simulink model "robot_4DOF_jointspace"  (Simulink 7.3)
settings: Solver=ode4  StartTime=0.0  StopTime=5  FixedStep=.002  MinStep=.002  RelTol=1e-3
libraries: simulink_extras x1, dspinverses x1
(part 1 of 2)
settings Model: Creator=arash  LastModifiedBy=arash
settings SolverCC: ExtrapolationOrder=1

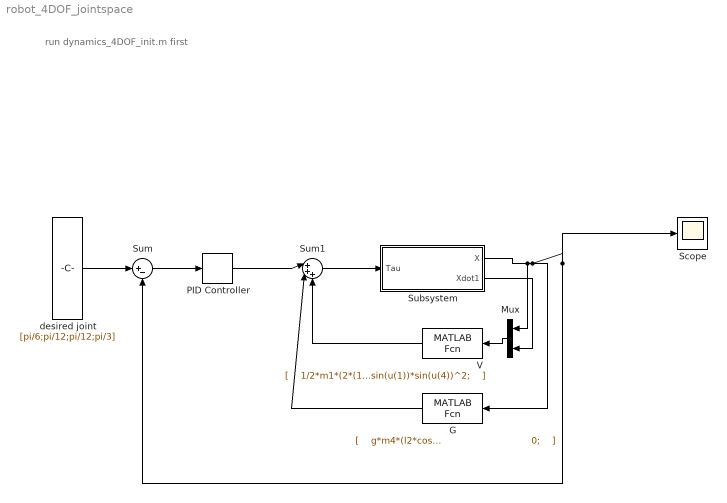
== system robot_4DOF_jointspace ==
  note: run dynamics_4DOF_init.m first
  G : MATLABFcn  MATLABFcn=|  OutputDimensions=4  OutputSignalType=real  Output1D=off
      | [
      |  
      |  g*m4*(l2*cos(u(1) + u(2)) + l1*cos(u(1)) + 1/2*l3*cos(u(1) + u(2) + u(3))) + g*m3*(1/2*l2*cos(u(1) + u(2)) + l1*cos(u(1))) + 1/2*g*l1*m2*cos(u(1));
      |                                                          g*m4*(l2*cos(u(1) + u(2)) + 1/2*l3*cos(u(1) + u(2) + u(3))) + 1/2*g*l2*m3*cos(u(1) + u(2));
      |                                                                                                                 1/2*g*l3*m4*cos(u(1) + u(2) + u(3));
      |                                                                                                                                                   0;
      |  
      |  ]
  Mux : Mux  Inputs=2
  PID Controller : simulink_extras/Additional Linear/PID Controller  SystemSampleTime=-1  P=[60;50;40;40]*10  I=[0;0;0;0]  D=[10;7;7;6]*5
  Scope : Scope
      settings: YMin=-0.05  YMax=1.1
  Subsystem : Subsystem
  Sum : Sum  Inputs=|+-  OutDataType=fixdt(1, 16)  OutScaling=2^0
  Sum1 : Sum  Inputs=|+++  OutDataType=fixdt(1, 16)  OutScaling=2^0
  V : MATLABFcn  MATLABFcn=|  OutputDimensions=4  OutputSignalType=real  Output1D=off
      | [
      |  
      |  1/2*m1*(2*(1/2*l1*u(8)*sin(u(1))*sin(u(4)) - 1/2*l1*u(5)*cos(u(1))*cos(u(4)))*(1/2*l1*u(5)*cos(u(4))*sin(u(1)) + 1/2*l1*u(8)*cos(u(1))*sin(u(4))) - 2*(1/2*l1*u(5)*sin(u(1))*sin(u(4)) - 1/2*l1*u(8)*cos(u(1))*cos(u(4)))*(1/2*l1*u(5)*cos(u(1))*sin(u(4)) + 1/2*l1*u(8)*cos(u(4))*sin(u(1))) + 1/2*l1^2*u(5)^2*cos(u(1))*sin(u(1))) + 1/2*m2*(2*sin(u(4))*(1/2*l2*sin(u(1) + u(2)) + l1*sin(u(1)))*(sin(u(4))*(1/2*l2*cos(u(1) + u(2)) + l1*cos(u(1)))*u(8)^2 + 2*cos(u(4))*(l1*u(5)*sin(u(1)) + 1/2*l2*sin(u(1) + u(2))*(u(5) + u(6)))*u(8) + sin(u(4))*(1/2*l2*cos(u(1) + u(2))*(u(5) + u(6))^2 + l1*u(5)^2*cos(u(1)))) - 2*(1/2*l2*sin(u(1) + u(2))*(u(5) + u(6))^2 + l1*u(5)^2*sin(u(1)))*(1/2*l2*cos(u(1) + u(2)) + l1*cos(u(1))) - 2*(l1*u(5)*cos(u(1)) + 1/2*l2*cos(u(1) + u(2))*(u(5) + u(6)))*(l1*u(5)*sin(u(1)) + 1/2*l2*sin(u(1) + u(2))*(u(5) + u(6))) + 2*cos(u(4))*(cos(u(4))*(l1*u(5)*sin(u(1)) + 1/2*l2*sin(u(1) + u(2))*(u(5) + u(6))) + u(8)*sin(u(4))*(1/2*l2*cos(u(1) + u(2)) + l1*cos(u(1))))*(l1*u(5)*cos(u(1)) + 1/2*l2*cos(u(1) + u(2))*(u(5) + u(6))) + 2*sin(u(4))*(sin(u(4))*(l1*u(5)*sin(u(1)) + 1/2*l2*sin(u(1) + u(2))*(u(5) + u(6))) - u(8)*cos(u(4))*(1/2*l2*cos(u(1) + u(2)) + l1*cos(u(1))))*(l1*u(5)*cos(u(1)) + 1/2*l2*cos(u(1) + u(2))*(u(5) + u(6))) + 2*cos(u(4))*(1/2*l2*sin(u(1) + u(2)) + l1*sin(u(1)))*(cos(u(4))*(1/2*l2*cos(u(1) + u(2)) + l1*cos(u(1)))*u(8)^2 - 2*sin(u(4))*(l1*u(5)*sin(u(1)) + 1/2*l2*sin(u(1) + u(2))*(u(5) + u(6)))*u(8) + cos(u(4))*(1/2*l2*cos(u(1) + u(2))*(u(5) + u(6))^2 + l1*u(5)^2*cos(u(1)))) + 2*u(8)*cos(u(4))*(sin(u(4))*(l1*u(5)*sin(u(1)) + 1/2*l2*sin(u(1) + u(2))*(u(5) + u(6))) - u(8)*cos(u(4))*(1/2*l2*cos(u(1) + u(2)) + l1*cos(u(1))))*(1/2*l2*sin(u(1) + u(2)) + l1*sin(u(1))) - 2*u(8)*sin(u(4))*(cos(u(4))*(l1*u(5)*sin(u(1)) + 1/2*l2*sin(u(1) + u(2))*(u(5) + u(6))) + u(8)*sin(u(4))*(1/2*l2*cos(u(1) + u(2)) + l1*cos(u(1))))*(1/2*l2*sin(u(1) + u(2)) + l1*sin(u(1)))) + c1*u(5) - 1/2*m3*(2*(sin(u(4))*(l1*u(5)*cos(u(1)) + 1/2*l3*cos(u(1) + u(2) + u(3))*(u(5) + u(6) + u(7)) + l2*cos(u(1) + u(2))*(u(5) + u(6))) + u(8)*cos(u(4))*(l2*sin(u(1) + u(2)) + l1*sin(u(1)) + 1/2*l3*sin(u(1) + u(2) + u(3))))*(sin(u(4))*(l1*u(5)*sin(u(1)) + 1/2*l3*sin(u(1) + u(2) + u(3))*(u(5) + u(6) + u(7)) + l2*sin(u(1) + u(2))*(u(5) + u(6))) - u(8)*cos(u(4))*(l2*cos(u(1) + u(2)) + l1*cos(u(1)) + 1/2*l3*cos(u(1) + u(2) + u(3)))) - 2*(l1*u(5)*sin(u(1)) + 1/2*l3*sin(u(1) + u(2) + u(3))*(u(5) + u(6) + u(7)) + l2*sin(u(1) + u(2))*(u(5) + u(6)))*(l1*u(5)*cos(u(1)) + 1/2*l3*cos(u(1) + u(2) + u(3))*(u(5) + u(6) + u(7)) + l2*cos(u(1) + u(2))*(u(5) + u(6))) + 2*(cos(u(4))*(l1*u(5)*sin(u(1)) + 1/2*l3*sin(u(1) + u(2) + u(3))*(u(5) + u(6) + u(7)) + l2*sin(u(1) + u(2))*(u(5) + u(6))) + u(8)*sin(u(4))*(l2*cos(u(1) + u(2)) + l1*cos(u(1)) + 1/2*l3*cos(u(1) + u(2) + u(3))))*(cos(u(4))*(l1*u(5)*cos(u(1)) + 1/2*l3*cos(u(1) + u(2) + u(3))*(u(5) + u(6) + u(7)) + l2*cos(u(1) + u(2))*(u(5) + u(6))) - u(8)*sin(u(4))*(l2*sin(u(1) + u(2)) + l1*sin(u(1)) + 1/2*l3*sin(u(1) + u(2) + u(3))))) - 1/2*m2*(2*(sin(u(4))*(l1*u(5)*cos(u(1)) + 1/2*l2*cos(u(1) + u(2))*(u(5) + u(6))) + u(8)*cos(u(4))*(1/2*l2*sin(u(1) + u(2)) + l1*sin(u(1))))*(sin(u(4))*(l1*u(5)*sin(u(1)) + 1/2*l2*sin(u(1) + u(2))*(u(5) + u(6))) - u(8)*cos(u(4))*(1/2*l2*cos(u(1) + u(2)) + l1*cos(u(1)))) + 2*(cos(u(4))*(l1*u(5)*sin(u(1)) + 1/2*l2*sin(u(1) + u(2))*(u(5) + u(6))) + u(8)*sin(u(4))*(1/2*l2*cos(u(1) + u(2)) + l1*cos(u(1))))*(cos(u(4))*(l1*u(5)*cos(u(1)) + 1/2*l2*cos(u(1) + u(2))*(u(5) + u(6))) - u(8)*sin(u(4))*(1/2*l2*sin(u(1) + u(2)) + l1*sin(u(1)))) - 2*(l1*u(5)*cos(u(1)) + 1/2*l2*cos(u(1) + u(2))*(u(5) + u(6)))*(l1*u(5)*sin(u(1)) + 1/2*l2*sin(u(1) + u(2))*(u(5) + u(6)))) + 1/2*m3*(2*cos(u(4))*(l2*sin(u(1) + u(2)) + l1*sin(u(1)) + 1/2*l3*sin(u(1) + u(2) + u(3)))*(cos(u(4))*(l2*cos(u(1) + u(2)) + l1*cos(u(1)) + 1/2*l3*cos(u(1) + u(2) + u(3)))*u(8)^2 - 2*sin(u(4))*(l1*u(5)*sin(u(1)) + 1/2*l3*sin(u(1) + u(2) + u(3))*(u(5) + u(6) + u(7)) + l2*sin(u(1) + u(2))*(u(5) + u(6)))*u(8) + cos(u(4))*(1/2*l3*cos(u(1) + u(2) + u(3))*(u(5) + u(6) + u(7))^2 + l2*cos(u(1) + u(2))*(u(5) + u(6))^2 + l1*u(5)^2*cos(u(1)))) - 2*(1/2*l3*sin(u(1) + u(2) + u(3))*(u(5) + u(6) + u(7))^2 + l2*sin(u(1) + u(2))*(u(5) + u(6))^2 + l1*u(5)^2*sin(u(1)))*(l2*cos(u(1) + u(2)) + l1*cos(u(1)) + 1/2*l3*cos(u(1) + u(2) + u(3))) - 2*(l1*u(5)*sin(u(1)) + 1/2*l3*sin(u(1) + u(2) + u(3))*(u(5) + u(6) + u(7)) + l2*sin(u(1) + u(2))*(u(5) + u(6)))*(l1*u(5)*cos(u(1)) + 1/2*l3*cos(u(1) + u(2) + u(3))*(u(5) + u(6) + u(7)) + l2*cos(u(1) + u(2))*(u(5) + u(6))) + 2*sin(u(4))*(l2*sin(u(1) + u(2)) + l1*sin(u(1)) + 1/2*l3*sin(u(1) + u(2) + u(3)))*(sin(u(4))*(l2*cos(u(1) + u(2)) + l1*cos(u(1)) + 1/2*l3*cos(u(1) + u(2) + u(3)))*u(8)^2 + 2*cos(u(4))*(l1*u(5)*sin(u(1)) + 1/2*l3*sin(u(1) + u(2) + u(3))*(u(5) + u(6) + u(7)) + l2*sin(u(1) + u(2))*(u(5) + u(6)))*u(8) + sin(u(4))*(1/2*l3*cos(u(1) + u(2) + u(3))*(u(5) + u(6) + u(7))^2 + l2*cos(u(1) + u(2))*(u(5) + u(6))^2 + l1*u(5)^2*cos(u(1)))) + 2*cos(u(4))*(cos(u(4))*(l1*u(5)*sin(u(1)) + 1/2*l3*sin(u(1) + u(2) + u(3))*(u(5) + u(6) + u(7)) + l2*sin(u(1) + u(2))*(u(5) + u(6))) + u(8)*sin(u(4))*(l2*cos(u(1) + u(2)) + l1*cos(u(1)) + 1/2*l3*cos(u(1) + u(2) + u(3))))*(l1*u(5)*cos(u(1)) + 1/2*l3*cos(u(1) + u(2) + u(3))*(u(5) + u(6) + u(7)) + l2*cos(u(1) + u(2))*(u(5) + u(6))) + 2*sin(u(4))*(sin(u(4))*(l1*u(5)*sin(u(1)) + 1/2*l3*sin(u(1) + u(2) + u(3))*(u(5) + u(6) + u(7)) + l2*sin(u(1) + u(2))*(u(5) + u(6))) - u(8)*cos(u(4))*(l2*cos(u(1) + u(2)) + l1*cos(u(1)) + 1/2*l3*cos(u(1) + u(2) + u(3))))*(l1*u(5)*cos(u(1)) + 1/2*l3*cos(u(1) + u(2) + u(3))*(u(5) + u(6) + u(7)) + l2*cos(u(1) + u(2))*(u(5) + u(6))) + 2*u(8)*cos(u(4))*(sin(u(4))*(l1*u(5)*sin(u(1)) + 1/2*l3*sin(u(1) + u(2) + u(3))*(u(5) + u(6) + u(7)) + l2*sin(u(1) + u(2))*(u(5) + u(6))) - u(8)*cos(u(4))*(l2*cos(u(1) + u(2)) + l1*cos(u(1)) + 1/2*l3*cos(u(1) + u(2) + u(3))))*(l2*sin(u(1) + u(2)) + l1*sin(u(1)) + 1/2*l3*sin(u(1) + u(2) + u(3))) - 2*u(8)*sin(u(4))*(cos(u(4))*(l1*u(5)*sin(u(1)) + 1/2*l3*sin(u(1) + u(2) + u(3))*(u(5) + u(6) + u(7)) + l2*sin(u(1) + u(2))*(u(5) + u(6))) + u(8)*sin(u(4))*(l2*cos(u(1) + u(2)) + l1*cos(u(1)) + 1/2*l3*cos(u(1) + u(2) + u(3))))*(l2*sin(u(1) + u(2)) + l1*sin(u(1)) + 1/2*l3*sin(u(1) + u(2) + u(3)))) + Ixx1*u(8)^2*cos(u(1))*sin(u(1)) - Izz1*u(8)^2*cos(u(1))*sin(u(1)) + Ixx3*u(8)^2*cos(u(1) + u(2) + u(3))*sin(u(1) + u(2) + u(3)) - Izz3*u(8)^2*cos(u(1) + u(2) + u(3))*sin(u(1) + u(2) + u(3)) + Ixx2*u(8)^2*cos(u(1) + u(2))*sin(u(1) + u(2)) - Izz2*u(8)^2*cos(u(1) + u(2))*sin(u(1) + u(2));
      |                                                                                                                                                                                                                                                                                                                                                                                                                                                                                                                                                                                                                                                                                                                                                                                                                                                                                                                                                                                                                                                                                                                                                                                                                                                                                                                                                                                                                                                                                                                                                                                                                                                                                                                                                                                                                                                                                                                                                                                                                                                                                                                                                                                                                                                                                                                                                                                                                                                                                                                                                                                                                                                                                                                                                                                                                                                                                                                                                                                                                                                                                                                                                                                                                                                                                                                                                                                                                                                                                                                                                                                                                                                                                                                                                                                                                                                                                                                                                                                                                                                                                                                                                                                                                                                                                                                                                                                                                                                                                                                                                                                                                                                                                                                                                                                                                                                                                                                                                                                                                                                                                       c2*u(6) - 1/2*m3*(2*(cos(u(4))*(l1*u(5)*sin(u(1)) + 1/2*l3*sin(u(1) + u(2) + u(3))*(u(5) + u(6) + u(7)) + l2*sin(u(1) + u(2))*(u(5) + u(6))) + u(8)*sin(u(4))*(l2*cos(u(1) + u(2)) + l1*cos(u(1)) + 1/2*l3*cos(u(1) + u(2) + u(3))))*(cos(u(4))*(1/2*l3*cos(u(1) + u(2) + u(3))*(u(5) + u(6) + u(7)) + l2*cos(u(1) + u(2))*(u(5) + u(6))) - u(8)*sin(u(4))*(l2*sin(u(1) + u(2)) + 1/2*l3*sin(u(1) + u(2) + u(3)))) + 2*(sin(u(4))*(l1*u(5)*sin(u(1)) + 1/2*l3*sin(u(1) + u(2) + u(3))*(u(5) + u(6) + u(7)) + l2*sin(u(1) + u(2))*(u(5) + u(6))) - u(8)*cos(u(4))*(l2*cos(u(1) + u(2)) + l1*cos(u(1)) + 1/2*l3*cos(u(1) + u(2) + u(3))))*(sin(u(4))*(1/2*l3*cos(u(1) + u(2) + u(3))*(u(5) + u(6) + u(7)) + l2*cos(u(1) + u(2))*(u(5) + u(6))) + u(8)*cos(u(4))*(l2*sin(u(1) + u(2)) + 1/2*l3*sin(u(1) + u(2) + u(3)))) - 2*(1/2*l3*sin(u(1) + u(2) + u(3))*(u(5) + u(6) + u(7)) + l2*sin(u(1) + u(2))*(u(5) + u(6)))*(l1*u(5)*cos(u(1)) + 1/2*l3*cos(u(1) + u(2) + u(3))*(u(5) + u(6) + u(7)) + l2*cos(u(1) + u(2))*(u(5) + u(6)))) - 1/2*m2*(2*(cos(u(4))*(l1*u(5)*sin(u(1)) + 1/2*l2*sin(u(1) + u(2))*(u(5) + u(6))) + u(8)*sin(u(4))*(1/2*l2*cos(u(1) + u(2)) + l1*cos(u(1))))*(1/2*l2*cos(u(1) + u(2))*cos(u(4))*(u(5) + u(6)) - 1/2*l2*u(8)*sin(u(1) + u(2))*sin(u(4))) + 2*(sin(u(4))*(l1*u(5)*sin(u(1)) + 1/2*l2*sin(u(1) + u(2))*(u(5) + u(6))) - u(8)*cos(u(4))*(1/2*l2*cos(u(1) + u(2)) + l1*cos(u(1))))*(1/2*l2*cos(u(1) + u(2))*sin(u(4))*(u(5) + u(6)) + 1/2*l2*u(8)*sin(u(1) + u(2))*cos(u(4))) - l2*sin(u(1) + u(2))*(l1*u(5)*cos(u(1)) + 1/2*l2*cos(u(1) + u(2))*(u(5) + u(6)))*(u(5) + u(6))) + Ixx3*u(8)^2*cos(u(1) + u(2) + u(3))*sin(u(1) + u(2) + u(3)) - Izz3*u(8)^2*cos(u(1) + u(2) + u(3))*sin(u(1) + u(2) + u(3)) + Ixx2*u(8)^2*cos(u(1) + u(2))*sin(u(1) + u(2)) - Izz2*u(8)^2*cos(u(1) + u(2))*sin(u(1) + u(2)) - 1/2*l2*l3*m3*u(7)^2*sin(u(3)) - 1/2*l1*l3*m3*u(5)*u(6)*sin(u(2) + u(3)) - 1/2*l1*l3*m3*u(5)*u(7)*sin(u(2) + u(3)) - 1/2*l1*l2*m2*u(5)*u(6)*sin(u(2)) - l1*l2*m3*u(5)*u(6)*sin(u(2)) - l2*l3*m3*u(5)*u(7)*sin(u(3)) - l2*l3*m3*u(6)*u(7)*sin(u(3));
      |                                                                                                                                                                                                                                                                                                                                                                                                                                                                                                                                                                                                                                                                                                                                                                                                                                                                                                                                                                                                                                                                                                                                                                                                                                                                                                                                                                                                                                                                                                                                                                                                                                                                                                                                                                                                                                                                                                                                                                                                                                                                                                                                                                                                                                                                                                                                                                                                                                                                                                                                                                                                                                                                                                                                                                                                                                                                                                                                                                                                                                                                                                                                                                                                                                                                                                                                                                                                                                                                                                                                                                                                                                                                                                                                                                                                                                                                                                                                                                                                                                                                                                                                                                                                                                                                                                                                                                                                                                                                                                                                                                                                                                                                                                                                                                                                                                                                                                                                                                                                                                                                                                                                                                                                                                                                                                                                                                                                                                                                                                                                                                                                                                                                                                                                                                                                                                                                                                                                                                                                                                                                                                                                    c3*u(7) + 1/2*m3*(2*(1/2*l3*u(8)*sin(u(1) + u(2) + u(3))*sin(u(4)) - 1/2*l3*cos(u(1) + u(2) + u(3))*cos(u(4))*(u(5) + u(6) + u(7)))*(cos(u(4))*(l1*u(5)*sin(u(1)) + 1/2*l3*sin(u(1) + u(2) + u(3))*(u(5) + u(6) + u(7)) + l2*sin(u(1) + u(2))*(u(5) + u(6))) + u(8)*sin(u(4))*(l2*cos(u(1) + u(2)) + l1*cos(u(1)) + 1/2*l3*cos(u(1) + u(2) + u(3)))) - 2*(1/2*l3*u(8)*sin(u(1) + u(2) + u(3))*cos(u(4)) + 1/2*l3*cos(u(1) + u(2) + u(3))*sin(u(4))*(u(5) + u(6) + u(7)))*(sin(u(4))*(l1*u(5)*sin(u(1)) + 1/2*l3*sin(u(1) + u(2) + u(3))*(u(5) + u(6) + u(7)) + l2*sin(u(1) + u(2))*(u(5) + u(6))) - u(8)*cos(u(4))*(l2*cos(u(1) + u(2)) + l1*cos(u(1)) + 1/2*l3*cos(u(1) + u(2) + u(3)))) + l3*sin(u(1) + u(2) + u(3))*(u(5) + u(6) + u(7))*(l1*u(5)*cos(u(1)) + 1/2*l3*cos(u(1) + u(2) + u(3))*(u(5) + u(6) + u(7)) + l2*cos(u(1) + u(2))*(u(5) + u(6)))) + Ixx3*u(8)^2*cos(u(1) + u(2) + u(3))*sin(u(1) + u(2) + u(3)) - Izz3*u(8)^2*cos(u(1) + u(2) + u(3))*sin(u(1) + u(2) + u(3)) - 1/2*l1*l3*m3*u(5)*u(6)*sin(u(2) + u(3)) - 1/2*l1*l3*m3*u(5)*u(7)*sin(u(2) + u(3)) - 1/2*l2*l3*m3*u(5)*u(7)*sin(u(3)) - 1/2*l2*l3*m3*u(6)*u(7)*sin(u(3));
      |                                                                                                                                                                                                                                                                                                                                                                                                                                                                                                                                                                                                                                                                                                                                                                                                                                                                                                                                                                                                                                                                                                                                                                                                                                                                                                                                                                                                                                                                                                                                                                                                                                                                                                                                                                                                                                                                                                                                                                                                                                                                                                                                                                                                                                                                                                                                                                                                                                                                                                                                                                                                                                                                                                                                                                                                                                                                                1/2*m2*(2*cos(u(4))*(sin(u(4))*(l1*u(5)*sin(u(1)) + 1/2*l2*sin(u(1) + u(2))*(u(5) + u(6))) - u(8)*cos(u(4))*(1/2*l2*cos(u(1) + u(2)) + l1*cos(u(1))))*(l1*u(5)*sin(u(1)) + 1/2*l2*sin(u(1) + u(2))*(u(5) + u(6))) - 2*sin(u(4))*(cos(u(4))*(l1*u(5)*sin(u(1)) + 1/2*l2*sin(u(1) + u(2))*(u(5) + u(6))) + u(8)*sin(u(4))*(1/2*l2*cos(u(1) + u(2)) + l1*cos(u(1))))*(l1*u(5)*sin(u(1)) + 1/2*l2*sin(u(1) + u(2))*(u(5) + u(6))) - 2*cos(u(4))*(1/2*l2*cos(u(1) + u(2)) + l1*cos(u(1)))*(sin(u(4))*(1/2*l2*cos(u(1) + u(2)) + l1*cos(u(1)))*u(8)^2 + 2*cos(u(4))*(l1*u(5)*sin(u(1)) + 1/2*l2*sin(u(1) + u(2))*(u(5) + u(6)))*u(8) + sin(u(4))*(1/2*l2*cos(u(1) + u(2))*(u(5) + u(6))^2 + l1*u(5)^2*cos(u(1)))) + 2*sin(u(4))*(1/2*l2*cos(u(1) + u(2)) + l1*cos(u(1)))*(cos(u(4))*(1/2*l2*cos(u(1) + u(2)) + l1*cos(u(1)))*u(8)^2 - 2*sin(u(4))*(l1*u(5)*sin(u(1)) + 1/2*l2*sin(u(1) + u(2))*(u(5) + u(6)))*u(8) + cos(u(4))*(1/2*l2*cos(u(1) + u(2))*(u(5) + u(6))^2 + l1*u(5)^2*cos(u(1)))) + 2*u(8)*cos(u(4))*(cos(u(4))*(l1*u(5)*sin(u(1)) + 1/2*l2*sin(u(1) + u(2))*(u(5) + u(6))) + u(8)*sin(u(4))*(1/2*l2*cos(u(1) + u(2)) + l1*cos(u(1))))*(1/2*l2*cos(u(1) + u(2)) + l1*cos(u(1))) + 2*u(8)*sin(u(4))*(sin(u(4))*(l1*u(5)*sin(u(1)) + 1/2*l2*sin(u(1) + u(2))*(u(5) + u(6))) - u(8)*cos(u(4))*(1/2*l2*cos(u(1) + u(2)) + l1*cos(u(1))))*(1/2*l2*cos(u(1) + u(2)) + l1*cos(u(1)))) + 1/2*m3*(2*cos(u(4))*(sin(u(4))*(l1*u(5)*sin(u(1)) + 1/2*l3*sin(u(1) + u(2) + u(3))*(u(5) + u(6) + u(7)) + l2*sin(u(1) + u(2))*(u(5) + u(6))) - u(8)*cos(u(4))*(l2*cos(u(1) + u(2)) + l1*cos(u(1)) + 1/2*l3*cos(u(1) + u(2) + u(3))))*(l1*u(5)*sin(u(1)) + 1/2*l3*sin(u(1) + u(2) + u(3))*(u(5) + u(6) + u(7)) + l2*sin(u(1) + u(2))*(u(5) + u(6))) - 2*sin(u(4))*(cos(u(4))*(l1*u(5)*sin(u(1)) + 1/2*l3*sin(u(1) + u(2) + u(3))*(u(5) + u(6) + u(7)) + l2*sin(u(1) + u(2))*(u(5) + u(6))) + u(8)*sin(u(4))*(l2*cos(u(1) + u(2)) + l1*cos(u(1)) + 1/2*l3*cos(u(1) + u(2) + u(3))))*(l1*u(5)*sin(u(1)) + 1/2*l3*sin(u(1) + u(2) + u(3))*(u(5) + u(6) + u(7)) + l2*sin(u(1) + u(2))*(u(5) + u(6))) - 2*cos(u(4))*(l2*cos(u(1) + u(2)) + l1*cos(u(1)) + 1/2*l3*cos(u(1) + u(2) + u(3)))*(sin(u(4))*(l2*cos(u(1) + u(2)) + l1*cos(u(1)) + 1/2*l3*cos(u(1) + u(2) + u(3)))*u(8)^2 + 2*cos(u(4))*(l1*u(5)*sin(u(1)) + 1/2*l3*sin(u(1) + u(2) + u(3))*(u(5) + u(6) + u(7)) + l2*sin(u(1) + u(2))*(u(5) + u(6)))*u(8) + sin(u(4))*(1/2*l3*cos(u(1) + u(2) + u(3))*(u(5) + u(6) + u(7))^2 + l2*cos(u(1) + u(2))*(u(5) + u(6))^2 + l1*u(5)^2*cos(u(1)))) + 2*sin(u(4))*(l2*cos(u(1) + u(2)) + l1*cos(u(1)) + 1/2*l3*cos(u(1) + u(2) + u(3)))*(cos(u(4))*(l2*cos(u(1) + u(2)) + l1*cos(u(1)) + 1/2*l3*cos(u(1) + u(2) + u(3)))*u(8)^2 - 2*sin(u(4))*(l1*u(5)*sin(u(1)) + 1/2*l3*sin(u(1) + u(2) + u(3))*(u(5) + u(6) + u(7)) + l2*sin(u(1) + u(2))*(u(5) + u(6)))*u(8) + cos(u(4))*(1/2*l3*cos(u(1) + u(2) + u(3))*(u(5) + u(6) + u(7))^2 + l2*cos(u(1) + u(2))*(u(5) + u(6))^2 + l1*u(5)^2*cos(u(1)))) + 2*u(8)*cos(u(4))*(cos(u(4))*(l1*u(5)*sin(u(1)) + 1/2*l3*sin(u(1) + u(2) + u(3))*(u(5) + u(6) + u(7)) + l2*sin(u(1) + u(2))*(u(5) + u(6))) + u(8)*sin(u(4))*(l2*cos(u(1) + u(2)) + l1*cos(u(1)) + 1/2*l3*cos(u(1) + u(2) + u(3))))*(l2*cos(u(1) + u(2)) + l1*cos(u(1)) + 1/2*l3*cos(u(1) + u(2) + u(3))) + 2*u(8)*sin(u(4))*(sin(u(4))*(l1*u(5)*sin(u(1)) + 1/2*l3*sin(u(1) + u(2) + u(3))*(u(5) + u(6) + u(7)) + l2*sin(u(1) + u(2))*(u(5) + u(6))) - u(8)*cos(u(4))*(l2*cos(u(1) + u(2)) + l1*cos(u(1)) + 1/2*l3*cos(u(1) + u(2) + u(3))))*(l2*cos(u(1) + u(2)) + l1*cos(u(1)) + 1/2*l3*cos(u(1) + u(2) + u(3)))) + c4*u(8) - 2*Ixx3*u(8)*cos(u(1) + u(2) + u(3))*sin(u(1) + u(2) + u(3))*(u(5) + u(6) + u(7)) + 2*Izz3*u(8)*cos(u(1) + u(2) + u(3))*sin(u(1) + u(2) + u(3))*(u(5) + u(6) + u(7)) - 2*Ixx1*u(5)*u(8)*cos(u(1))*sin(u(1)) + 2*Izz1*u(5)*u(8)*cos(u(1))*sin(u(1)) - 2*Ixx2*u(8)*cos(u(1) + u(2))*sin(u(1) + u(2))*(u(5) + u(6)) + 2*Izz2*u(8)*cos(u(1) + u(2))*sin(u(1) + u(2))*(u(5) + u(6)) - 1/2*l1^2*m1*u(5)*u(8)*cos(u(1))*cos(u(4))^2*sin(u(1)) - 1/2*l1^2*m1*u(5)*u(8)*cos(u(1))*sin(u(1))*sin(u(4))^2;
      |  
      |  ]
  desired joint : Constant  Value=[pi/6;pi/12;pi/12;pi/3]  OutDataType=fixdt(1, 16)  OutScaling=2^0
  wires:
  desired joint/1 -> Sum/1
  Subsystem/1(X) -> Sum/2, Scope/1, G/1, Mux/1
  Sum/1 -> PID Controller/1
  Sum1/1 -> Subsystem/1(Tau)
  PID Controller/1 -> Sum1/1
  G/1 -> Sum1/2
  V/1 -> Sum1/3
  Mux/1 -> V/1
  Subsystem/2(Xdot1) -> Mux/2
